simulink model "EJERCICIO_1_MODIFICADO"  (Simulink 5.0)
settings: Solver=ode45  StartTime=0.0  StopTime=25.0  RelTol=1e-3
undefined symbols (not defined in the file): a, b, Gama, Km, Kp
settings Model: LastModifiedBy=Administrador

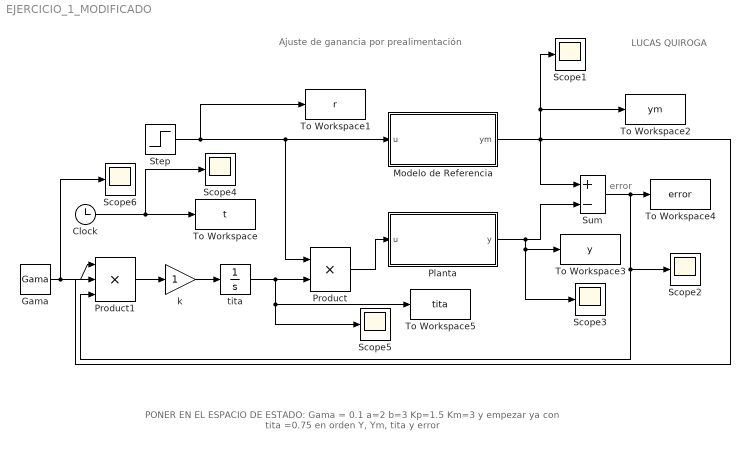
== system EJERCICIO_1_MODIFICADO ==
  note: error
  note: Ajuste de ganancia por prealimentación
  note: LUCAS QUIROGA
  note: PONER EN EL ESPACIO DE ESTADO:
      | Gama = 0.1
      | a=2
      | b=3
      | Kp=1.5
      | Km=3
      | y empezar ya con tita =0.75 en orden Y, Ym, tita y error
  Clock : Clock
      settings: Decimation=10
  Gama : Constant  Value=Gama
  Modelo de Referencia : Subsystem
  Planta : Subsystem
  Product : Product  SaturateOnIntegerOverflow=on
  Product1 : Product  Inputs=3  SaturateOnIntegerOverflow=on
  Scope{1..6} (6 alike) : Scope
      Scope1 settings: TimeRange=25  YMin=0
      Scope2 settings: TimeRange=25  YMin=0  YMax=2
      Scope3 settings: TimeRange=25  YMin=0  YMax=2  SaveName=ScopeData2
      Scope4 settings: TimeRange=25  YMin=0  YMax=2  SaveName=ScopeData4
      Scope5 settings: TimeRange=25  YMin=0  YMax=2  SaveName=ScopeData3
      Scope6 settings: TimeRange=25  YMin=0  YMax=0.005  SaveName=ScopeData5
  Step : Step  SampleTime=0
  Sum : Sum  Inputs=+-  SaturateOnIntegerOverflow=on
  To Workspace : ToWorkspace  VariableName=t  SampleTime=-1  SaveFormat=Array
  To Workspace1 : ToWorkspace  VariableName=r  SampleTime=-1  SaveFormat=Array
  To Workspace2 : ToWorkspace  VariableName=ym  SampleTime=-1  SaveFormat=Array
  To Workspace3 : ToWorkspace  VariableName=y  SampleTime=-1  SaveFormat=Array
  To Workspace4 : ToWorkspace  VariableName=error  SampleTime=-1  SaveFormat=Array
  To Workspace5 : ToWorkspace  VariableName=tita  SampleTime=-1  SaveFormat=Array
  k : Gain  SaturateOnIntegerOverflow=on
  tita : Integrator
  wires:
  Clock/1 -> To Workspace/1, Scope4/1
  Step/1 -> To Workspace1/1, Product/1, Modelo de Referencia/1(u)
  Modelo de Referencia/1(ym) -> Sum/1, Product1/2, To Workspace2/1, Scope1/1
  Planta/1(y) -> Sum/2, To Workspace3/1, Scope3/1
  Product/1 -> Planta/1(u)
  tita/1 -> Product/2, To Workspace5/1, Scope5/1
  k/1 -> tita/1
  Product1/1 -> k/1
  Gama/1 -> Product1/1, Scope6/1
  Sum/1 -> To Workspace4/1, Product1/3, Scope2/1

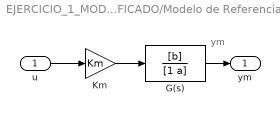
== system EJERCICIO_1_MODIFICADO/Modelo de Referencia ==
  note: ym
  u : Inport
  G(s) : TransferFcn  Numerator=[b]  Denominator=[1 a]
  Km : Gain  Gain=Km  SaturateOnIntegerOverflow=on
  ym : Outport
  wires:
  Km/1 -> G(s)/1
  u/1 -> Km/1
  G(s)/1 -> ym/1

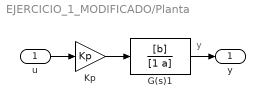
== system EJERCICIO_1_MODIFICADO/Planta ==
  note: y
  u : Inport
  G(s)1 : TransferFcn  Numerator=[b]  Denominator=[1 a]
  Kp : Gain  Gain=Kp  SaturateOnIntegerOverflow=on
  y : Outport
  wires:
  Kp/1 -> G(s)1/1
  G(s)1/1 -> y/1
  u/1 -> Kp/1
